simulink model "func"  (R2018a)
settings: Solver=FixedStepAuto  StartTime=0.0  StopTime=100  FixedStep=T  RelTol=1e-3
values from neighbouring files (symbols this model uses):
  Bt = 1e-3    (= 0.001)    [parameters.m]
  Jt = 0.055    [parameters.m]
  Lm = 0.1269    [asmodel.m]    (also in parameters.m = 0.135)
  Lr = Lm+Llr    (= 0.1443)    [asmodel.m]    (also in parameters.m = 0.1524)
  Lsigma = Ls-(Lm^2)/Lr    (= 0.0269018711019)    [asmodel.m]    (also in parameters.m = 0.0270133858268)
  Pp = 3    [asmodel.m]    (also in parameters.m)
  Rr = 2.53    [asmodel.m]    (also in parameters.m = 2.54)
  Rs = 3.03    [asmodel.m]    (also in dcmotor.m = 0.03; parameters.m = 3.04)
  T = 100e-6    (= 0.0001)    [asmodel.m]    (also in parameters.m)
  V_amp = 220*sqrt(2)    [parameters.m]
  we = 2*pi*50    (= 314.159265359)    [parameters.m]
settings Model: Creator=hp  LastModifiedBy=hp

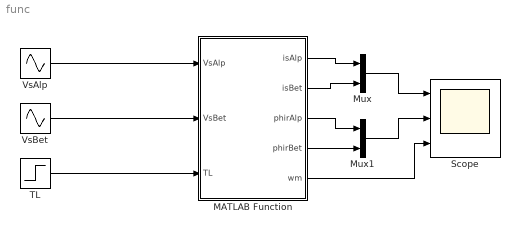
== system func ==
  MATLAB Function : MATLAB Function  TreatAsAtomicUnit=on
  Mux : Mux  Inputs=2
  Mux1 : Mux  Inputs=2
  Scope : Scope  NumInputPorts=3
  TL : Step  After=20  SampleTime=0
  "VsAlp " : Sin  Amplitude=V_amp  Frequency=we  Phase=pi/2  SampleTime=0
  "VsBet " : Sin  Amplitude=V_amp  Frequency=we  SampleTime=0
  wires:
  "VsAlp "/1 -> MATLAB Function/1(VsAlp)
  "VsBet "/1 -> MATLAB Function/2(VsBet)
  TL/1 -> MATLAB Function/3(TL)
  MATLAB Function/3(phirAlp) -> Mux1/1
  MATLAB Function/4(phirBet) -> Mux1/2
  MATLAB Function/2(isBet) -> Mux/2
  MATLAB Function/1(isAlp) -> Mux/1
  Mux1/1 -> Scope/2
  Mux/1 -> Scope/1
  MATLAB Function/5(wm) -> Scope/3

== matlab function func/MATLAB Function ==
  data: VsAlp input; isAlp output; VsBet input; TL input; isBet output; phirAlp output; phirBet output; wm output; Rs parameter; Lsigma parameter; Rr parameter; Lm parameter; Lr parameter; Bt parameter; Jt parameter; T parameter; Pp parameter

function [isAlp, isBet, phirAlp, phirBet,wm] = IMmodel(VsAlp, VsBet,TL, Rs, Lsigma, Rr, Lm, Lr, Bt, Jt, T, Pp)

persistent IsAlp IsBet PhirAlp PhirBet Wm

if isempty(IsAlp)
IsAlp=0;
IsBet =0;
PhirAlp = 0;
PhirBet =0;
Wm = 0;
end

isAlp = (1-(Rs/Lsigma+Lm^2*Rr/(Lsigma*Lr^2))*T)*IsAlp + Lm *Rr*T*PhirAlp /(Lsigma* Lr^2) + Lm+Pp*Wm* T* PhirBet/(Lsigma*Lr) + T*VsAlp/ Lsigma;

isBet = (1-(Rs/Lsigma+Lm^2*Rr/(Lsigma*Lr^2))*T)*IsBet + Lm *Rr*T*PhirBet /(Lsigma* Lr^2) - Lm+Pp*Wm* T* PhirAlp/(Lsigma*Lr) + T*VsBet/ Lsigma;

phirAlp = Rr*Lm*T*IsAlp/Lr + (1-Rr*T/Lr) * PhirAlp - Pp *Wm *T *PhirBet;

phirBet = Rr*Lm*T*IsBet/Lr + (1-Rr*T/Lr) * PhirBet - Pp *Wm *T *PhirAlp;

wm= (3*Pp * Lm/ (Jt * Lr)) * (PhirAlp*IsBet-PhirBet*IsAlp)*T + (1-Bt*T/Jt)*Wm - TL*T/Jt;

IsAlp= isAlp;  IsBet = isBet; PhirAlp = phirAlp; PhirBet=phirBet; Wm=wm;
